simulink model "RC_values"  (Simulink 8.9)
settings: Solver=ode45  StartTime=0.0  StopTime=10.0  RelTol=1e-3  EnableMultiTasking=on
settings Model: SuppressorTable=22 serialization::archive 11 0 6 0 0 0 0 0  Creator=hlopez5  LastModifiedBy=judithlopez
settings DataIOCC: SignalLoggingSaveFormat=Dataset
settings DebuggingCC: UnderspecifiedInitializationDetection=Simplified  MergeDetectMultiDrivingBlocksExec=error  FcnCallInpInsideContextMsg=error
settings GRTTargetCC: CombineOutputUpdateFcns=on  GRTInterface=off

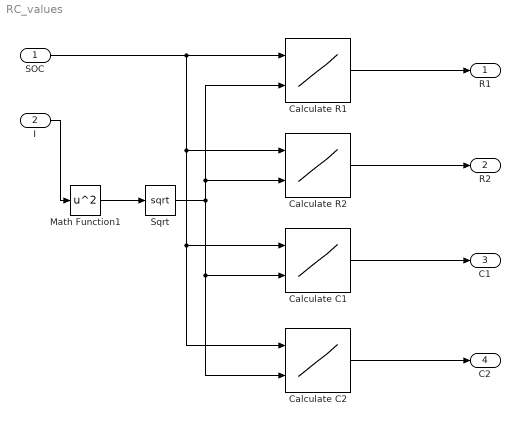
== system RC_values ==
  "SOC " : Inport
  I : Inport  Port=2
  Calculate C1 : Lookup_n-D  BreakpointsForDimension1=[1:3]  BreakpointsForDimension2=[1:3]  RndMeth=Simplest  InputSameDT=on
  Calculate C2 : Lookup_n-D  BreakpointsForDimension1=[1:3]  BreakpointsForDimension2=[1:3]  RndMeth=Simplest  InputSameDT=on
  Calculate R1 : Lookup_n-D  BreakpointsForDimension1=[1,2,3]  BreakpointsForDimension2=[1,2,3]  Table=reshape([21.2303,5.7784,4.3207,22.9213,6.8863,4.0875,23.2128,6.7697,4.0292],3,3)  RndMeth=Simplest  InputSameDT=on
  Calculate R2 : Lookup_n-D  BreakpointsForDimension1=[1,2,3]  BreakpointsForDimension2=[1,2,3]  Table=reshape([21.0292,5.3382,4.3207,19.7697,4.7609,4.4373,21.9883,6.1866,4.4461],3,3)  RndMeth=Simplest  InputSameDT=on
  Math Function1 : Math  Operator=square  SaturateOnIntegerOverflow=on
  Sqrt : Sqrt  SaturateOnIntegerOverflow=on
  R1 : Outport
  R2 : Outport  Port=2
  C1 : Outport  Port=3
  C2 : Outport  Port=4
  wires:
  I/1 -> Math Function1/1
  Math Function1/1 -> Sqrt/1
  Calculate R1/1 -> R1/1
  Calculate R2/1 -> R2/1
  Calculate C1/1 -> C1/1
  Calculate C2/1 -> C2/1
  Sqrt/1 -> Calculate R2/2, Calculate R1/2, Calculate C2/2, Calculate C1/2
  "SOC "/1 -> Calculate C2/1, Calculate C1/1, Calculate R2/1, Calculate R1/1
